simulink model "TestingPins"  (R2020a)
settings: Solver=ode4  StartTime=0.0  StopTime=7200  FixedStep=0.1  RelTol=1e-3  EnableMultiTasking=on
libraries: raspberrypiBasiclib x10, embdlinuxlib x3, sensehatlib x2, mspfiltlib x1
settings Model: ExtModeTrigDuration=2  Creator=AlexC  LastModifiedBy=AlexC
settings SolverCC: PositivePriorityOrder=on
settings DataIOCC: ReturnWorkspaceOutputs=off
settings OptimizationCC: MaxStackSize=64
settings DebuggingCC: MultiTaskDSMMsg=none  ParameterTunabilityLossMsg=error  ArithmeticOperatorsInVariantConditions=warning
settings HardwareCC: ProdBitPerPointer=32  ProdBitPerSizeT=32  ProdBitPerPtrDiffT=32  ProdLargestAtomicInteger=Long  ProdLargestAtomicFloat=Double  ProdWordSize=32  ProdLongLongMode=on  ProdHWDeviceType=ARM Compatible->ARM Cortex
settings SFSimCC: SimUseLocalCustomCode=off  CustomCodeUndefinedFunction=UseInterfaceOnly
settings RTWCC: SystemTargetFile=ert.tlc  HardwareBoard=Raspberry Pi  TemplateMakefile=ert_default_tmf  RTWUseLocalCustomCode=off  Toolchain=GNU GCC Raspberry Pi  BuildConfiguration=Faster Runs  TargetLang=C++
settings CodeAppCC: ForceParamTrailComments=on  OperatorAnnotations=on  StateflowObjectComments=on  MATLABSourceComments=on
settings ERTTargetCC: ERTCustomFileBanners=off  MatFileLogging=on  SupportContinuousTime=on  SupportNonInlinedSFcns=on  RemoveResetFunc=off  SupportVariableSizeSignals=on  ModelStepFunctionPrototypeControlCompliant=off

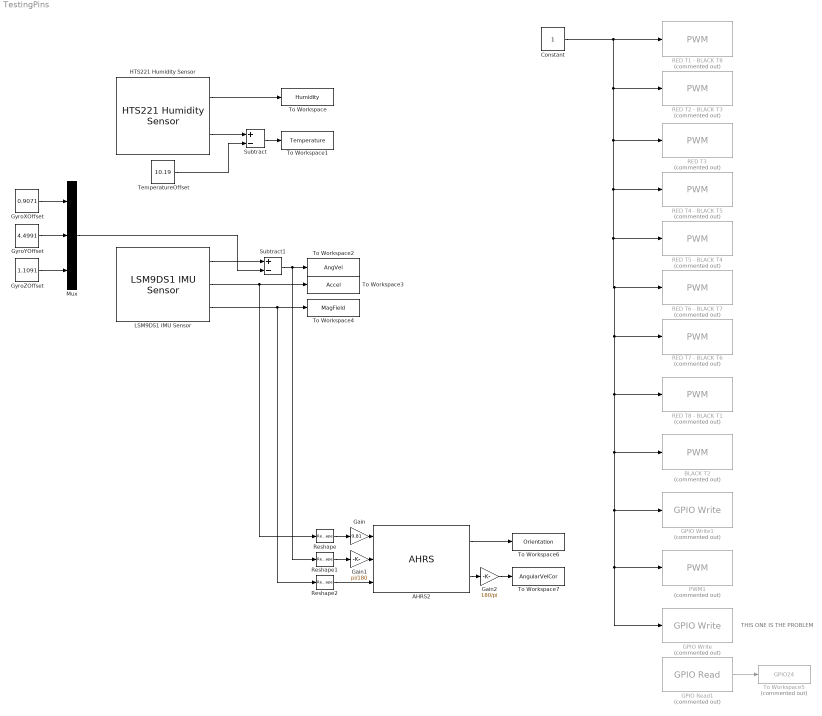
== system TestingPins ==
  note: THIS ONE IS THE PROBLEM
  AHRS2 : mspfiltlib/AHRS  DispRefFrame=NED  DecimationFactor=1  InitialProcessNoise=ahrsfilter.defaultProcessNoise  OrientationFormat=quaternion  SimulateUsing=Interpreted execution  AccelerometerNoise=0.0001924722  GyroscopeNoise=9.1385e-5  MagnetometerNoise=0.1  GyroscopeDriftNoise=3.0462e-13  LinearAccelerationNoise=0.0096236100000000012  MagneticDisturbanceNoise=0.5  LinearAccelerationDecayFactor=0.5  MagneticDisturbanceDecayFactor=0.5  ExpectedMagneticFieldStrength=33
      settings: SourceProductBaseCode=TF,NV
  BLACK T2 : raspberrypiBasiclib/PWM  Commented=on  board=Pi 3 Model B  Pin_=9  Frequency=10  blockPlatform=Raspberry Pi
      settings: SourceProductBaseCode=RASPPI
  Constant : Constant  VectorParams1D=off  SampleTime=-1
  GPIO Read1 : embdlinuxlib/GPIO Read  Commented=on  board=Pi 3 Model B  gpio=24  internalResistor=Off  sampleTime=0.1  direction=Input  blockPlatform=Raspberry Pi
      settings: SourceProductBaseCode=SC_BEAGLEBONE_BLUE,RASPPI
  GPIO Write : embdlinuxlib/GPIO Write  Commented=on  board=Pi 3 Model B  gpio=21  direction=Output  blockPlatform=Raspberry Pi
      settings: SourceProductBaseCode=SC_BEAGLEBONE_BLUE,RASPPI
  GPIO Write1 : embdlinuxlib/GPIO Write  Commented=on  board=Pi 3 Model B  gpio=25  direction=Output  blockPlatform=Raspberry Pi
      settings: SourceProductBaseCode=SC_BEAGLEBONE_BLUE,RASPPI
  Gain : Gain  Gain=9.81
  Gain1 : Gain  Gain=pi/180
  Gain2 : Gain  Gain=180/pi
  GyroXOffset : Constant  Value=0.9071  VectorParams1D=off  SampleTime=-1
  GyroYOffset : Constant  Value=4.4991  VectorParams1D=off  SampleTime=-1
  GyroZOffset : Constant  Value=1.1091  VectorParams1D=off  SampleTime=-1
  HTS221 Humidity Sensor : sensehatlib/HTS221 Humidity Sensor  BoardProperty=Pi 3 Model B  OutputDataRate=12.5 Hz  SampleTime=0.1
      settings: SourceProductBaseCode=RASPPI
  LSM9DS1 IMU Sensor : sensehatlib/LSM9DS1 IMU Sensor  blockPlatform=Raspberry Pi  BoardProperty_sh=Pi 3 Model B  ActiveSensors_=Accelerometer, Gyroscope and Magnetometer  AccelerometerOutputDataRate=119 Hz  AccelerometerFullScaleRange=+/- 2g  AccelerometerBandwidth=50 Hz  GyroscopeOutputDataRate=119 Hz  GyroscopeFullScaleRange=245 dps  GyroscopeBandwidthMode=0  GyroscopeHighPassFilterEnabled=off  GyroscopeHighPassFilterMode=0  MagnetometerFullScaleRange=+/- 4 gauss  MagnetometerOutputDataRate=40 Hz  SampleTime=0.1
      settings: SourceProductBaseCode=RASPPI
  Mux : Mux  Inputs=3
  PWM1 : raspberrypiBasiclib/PWM  Commented=on  board=Pi 3 Model B  Pin_=18  Frequency=10  blockPlatform=Raspberry Pi
      settings: SourceProductBaseCode=RASPPI
  RED T1 - BLACK T8 : raspberrypiBasiclib/PWM  Commented=on  board=Pi 3 Model B  Pin_=27  Frequency=10  blockPlatform=Raspberry Pi
      settings: SourceProductBaseCode=RASPPI
  RED T2 - BLACK T3 : raspberrypiBasiclib/PWM  Commented=on  board=Pi 3 Model B  Pin_=19  Frequency=10  blockPlatform=Raspberry Pi
      settings: SourceProductBaseCode=RASPPI
  RED T3 : raspberrypiBasiclib/PWM  Commented=on  board=Pi 3 Model B  Pin_=4  Frequency=10  blockPlatform=Raspberry Pi
      settings: SourceProductBaseCode=RASPPI
  RED T4 - BLACK T5 : raspberrypiBasiclib/PWM  Commented=on  board=Pi 3 Model B  Pin_=22  Frequency=10  blockPlatform=Raspberry Pi
      settings: SourceProductBaseCode=RASPPI
  RED T5 - BLACK T4 : raspberrypiBasiclib/PWM  Commented=on  board=Pi 3 Model B  Pin_=5  Frequency=10  blockPlatform=Raspberry Pi
      settings: SourceProductBaseCode=RASPPI
  RED T6 - BLACK T7 : raspberrypiBasiclib/PWM  Commented=on  board=Pi 3 Model B  Pin_=6  Frequency=10  blockPlatform=Raspberry Pi
      settings: SourceProductBaseCode=RASPPI
  RED T7 - BLACK T6 : raspberrypiBasiclib/PWM  Commented=on  board=Pi 3 Model B  Pin_=13  Frequency=10  blockPlatform=Raspberry Pi
      settings: SourceProductBaseCode=RASPPI
  RED T8 - BLACK T1 : raspberrypiBasiclib/PWM  Commented=on  board=Pi 3 Model B  Pin_=17  Frequency=10  blockPlatform=Raspberry Pi
      settings: SourceProductBaseCode=RASPPI
  Reshape : Reshape  OutputDimensionality=Row vector (2-D)
  Reshape1 : Reshape  OutputDimensionality=Row vector (2-D)
  Reshape2 : Reshape  OutputDimensionality=Row vector (2-D)
  Subtract : Sum  Inputs=+-
  Subtract1 : Sum  Inputs=+-
  TemperatureOffset : Constant  Value=10.19  VectorParams1D=off  SampleTime=-1
  To Workspace : ToWorkspace  VariableName=Humidity  SampleTime=-1
      settings: Save2DSignal=2-D array (concatenate along first dimension)
  To Workspace1 : ToWorkspace  VariableName=Temperature  SampleTime=-1
      settings: Save2DSignal=2-D array (concatenate along first dimension)
  To Workspace2 : ToWorkspace  VariableName=AngVel  SampleTime=-1
      settings: Save2DSignal=2-D array (concatenate along first dimension)
  To Workspace3 : ToWorkspace  VariableName=Accel  SampleTime=-1
      settings: Save2DSignal=2-D array (concatenate along first dimension)
  To Workspace4 : ToWorkspace  VariableName=MagField  SampleTime=-1
      settings: Save2DSignal=2-D array (concatenate along first dimension)
  To Workspace5 : ToWorkspace  Commented=on  VariableName=GPIO24  SampleTime=-1
      settings: Save2DSignal=2-D array (concatenate along first dimension)
  To Workspace6 : ToWorkspace  VariableName=Orientation  SampleTime=-1
      settings: Save2DSignal=2-D array (concatenate along first dimension)
  To Workspace7 : ToWorkspace  VariableName=AngularVelCor  SampleTime=-1
      settings: Save2DSignal=2-D array (concatenate along first dimension)
  wires:
  Constant/1 -> PWM1/1, GPIO Write/1, GPIO Write1/1, BLACK T2/1, RED T8 - BLACK T1/1, RED T7 - BLACK T6/1, RED T6 - BLACK T7/1, RED T5 - BLACK T4/1, RED T4 - BLACK T5/1, RED T3/1, RED T2 - BLACK T3/1, RED T1 - BLACK T8/1
  HTS221 Humidity Sensor/1 -> To Workspace/1
  GPIO Read1/1 -> To Workspace5/1
  Gain/1 -> AHRS2/1
  Gain1/1 -> AHRS2/2
  AHRS2/1 -> To Workspace6/1
  AHRS2/2 -> Gain2/1
  Gain2/1 -> To Workspace7/1
  HTS221 Humidity Sensor/2 -> Subtract/1
  Subtract/1 -> To Workspace1/1
  TemperatureOffset/1 -> Subtract/2
  Reshape/1 -> Gain/1
  Reshape2/1 -> AHRS2/3
  Reshape1/1 -> Gain1/1
  GyroXOffset/1 -> Mux/1
  GyroYOffset/1 -> Mux/2
  GyroZOffset/1 -> Mux/3
  LSM9DS1 IMU Sensor/1 -> Subtract1/1
  Mux/1 -> Subtract1/2
  Subtract1/1 -> Reshape1/1, To Workspace2/1
  LSM9DS1 IMU Sensor/2 -> Reshape/1, To Workspace3/1
  LSM9DS1 IMU Sensor/3 -> Reshape2/1, To Workspace4/1
